simulink model "MagneticBasket_Simscape_Optimizer"  (R2023b)
settings: Solver=VariableStepAuto  StartTime=0.0  StopTime=SimParams.SimulationTime  MaxStep=1e-3
values from neighbouring files (symbols this model uses):
  m = obj.Br *obj.volume / obj.mu    [External_Magnet2.m]
  W = 1.5e-3    (= 0.0015)    [Sim_Open.m]
  x = x + link_length * sin(current_angle)    [Robot_Kinematics.m]    (also in Run_SimOpt.m = [Input.DipoleMoment_Angle{Input.Index} Input.DipoleMoment_Ma; magnetic_robot_simulation_old.m = x + dx; optimize_magnetic_robot.m = x + dx; optimize_magnetic_robot_second.m = x + dx)
undefined symbols (not defined in the file or in its folder): Fixed, magnet_HomePosition, SimParams, X, Y, Z
libraries: sm_lib x87, nesl_utility x48, vrlib x32, matrix_library x16
(part 3 of 3)

== system MagneticBasket_Simscape_Optimizer/Subsystem1/Magnetic Torque//Force Generator6 ==
  Calculate Magnetic Force/Torque : Subsystem
  Display{,1..4} (5 alike) : Display
  External Force and Torque : sm_lib/Forces and Torques/External Force and Torque  ForceResolutionFrame=AttachedFrame  EnableForceX=off  EnableForceY=off  EnableForceZ=off  EnableForce=on  TorqueResolutionFrame=AttachedFrame  EnableTorqueX=off  EnableTorqueY=off  EnableTorqueZ=off  EnableTorque=on
  Gain1 : Gain  Gain=SimParams.force_onoff
  Gain2 : Gain  Gain=SimParams.torque_onoff
  Indexing Needed : Gain  Gain=x(13)
  Indexing Needed2 : sm_lib/Frames and Transforms/Rigid Transform  TranslationMethod=None  TranslationStandardOffset=0  TranslationStandardOffsetUnits=m  TranslationStandardAxis=+Z  TranslationCartesianOffset=[0 0 0]  TranslationCartesianOffsetUnits=m  TranslationROffset=0  TranslationROffsetUnits=m  TranslationZOffset=0  TranslationZOffsetUnits=m  TranslationThetaOffset=0  TranslationThetaOffsetUnits=deg  RotationMethod=StandardAxis  RotationAngleUnits=deg  RotationStandardAxis=-Y  RotationAngle=x(6)*180/pi-90  RotationArbitraryAxis=[0 0 1]  FollAlignAxisA=+X  BaseAlignAxisA=+Y  FollAlignAxisB=+Y  BaseAlignAxisB=+Z  RotationSequenceAxes=FollowerAxes  RotationSequence=YXZ  RotationSequenceAngles=[-90 -90 0]  RotationSequenceAnglesUnits=deg  RotationMatrix=[1 0 0; 0 1 0; 0 0 1]  Quaternion=[1 0 0 0]
  Indexing Needed3 : sm_lib/Body Elements/Cylindrical Solid  GraphicAmbientColor=[0.15 0.15 0.15 1.0]  BasedOnType=Density  CenterOfMass=[0 0 0]  CenterOfMassUnits=m  GraphicDiffuseColor=[1 0 0]  CylinderLength=1e4*SimParams.arrow_scale*x(13)  CylinderLengthUnits=mm  CylinderRadius=SimParams.arrow_scale*0.05  CylinderRadiusUnits=mm  Density=0  DensityUnits=kg/m^3  DoExposeReferenceFrame=off  GraphicEmissiveColor=[0.0 0.0 0.0 1.0]  ExportEntireGeometry=off  SerializedFrames=<Frames><Frame><Id>Frame1</Id><Value><Name>F1</Name><Origin><Source>GeometricFeature</Source><FeatureName>top surface</FeatureName></Origin><PrimaryAxis><DefinedDirection>+Z</DefinedDirection><Source>ReferenceFrame</Source><SourceDirection>+Z</SourceDirection><FeatureName></FeatureName></PrimaryAxis><SecondaryAxis><DefinedDirection>+X</DefinedDirection><Source>ReferenceFrame</Source><SourceDirection>+X</SourceDirection><FeatureName></FeatureName></SecondaryAxis></Value></Frame><Frame><Id>Frame2</Id><Value><Name>F2</Name><Origin><Source>GeometricFeature</Source><FeatureName>bottom surface</FeatureName></Origin><PrimaryAxis><DefinedDirection>+Z</DefinedDirection><Source>ReferenceFrame</Source><SourceDirection>+Z</SourceDirection><FeatureName></FeatureName></PrimaryAxis><SecondaryAxis><DefinedDirection>+X</DefinedDirection><Source>ReferenceFrame</Source><SourceDirection>+X</SourceDirection><FeatureName></FeatureName></SecondaryAxis></Value></Frame></Frames>  MarkerShape=Sphere  MarkerSize=10  GraphicType=FromGeometry  InertiaType=CalculateFromGeometry  Mass=1  MassUnits=kg  MomentsOfInertia=[1 1 1]  MomentsOfInertiaUnits=kg*m^2  GraphicOpacity=SimParams.arrow_Opacity  ProductsOfInertia=[0 0 0]  ProductsOfInertiaUnits=kg*m^2  GraphicShininess=75  GraphicSpecularColor=[0.5 0.5 0.5 1.0]  GraphicVisPropType=SimpleVisualProperties
  Magnet DipoleMoment : Constant  Value=[Fixed.MagnetDirection 0]*Fixed.MagnetMagnitude
  MatrixMultiply : Product  Multiplication=Matrix(*)
  Normalize Vector : vrlib/Utilities/Normalize Vector  maxzero=0
  PS-Simulink Converter1 : nesl_utility/PS-Simulink Converter  PhysicalDomain=network_engine_domain  SubClassName=ps_output  LeftPortType=input  RightPortType=output  PseudoPeriodic=off  Frequencies=[]  VectorFormat=inherit  Unit=inherit  AffineConversion=off
  PS-Simulink Converter2 : nesl_utility/PS-Simulink Converter  PhysicalDomain=network_engine_domain  SubClassName=ps_output  LeftPortType=input  RightPortType=output  PseudoPeriodic=off  Frequencies=[]  VectorFormat=inherit  Unit=inherit  AffineConversion=off
  PS-Simulink Converter3 : nesl_utility/PS-Simulink Converter  PhysicalDomain=network_engine_domain  SubClassName=ps_output  LeftPortType=input  RightPortType=output  PseudoPeriodic=off  Frequencies=[]  VectorFormat=inherit  Unit=inherit  AffineConversion=off
  Revolved Solid : sm_lib/Body Elements/Revolved Solid  GraphicAmbientColor=[0.15 0.15 0.15 1.0]  BasedOnType=Density  CenterOfMass=[0 0 0]  CenterOfMassUnits=m  GraphicDiffuseColor=[1.0 0.0 0]  ExportConvexHullGeometry=off  Density=0  DensityUnits=kg/m^3  DoExposeReferenceFrame=on  GraphicEmissiveColor=[0.0 0.0 0.0 1.0]  ExportEntireGeometry=off  SerializedFrames=<Frames/>  MarkerShape=Sphere  MarkerSize=10  GraphicType=FromGeometry  InertiaType=CalculateFromGeometry  Mass=1  MassUnits=kg  MomentsOfInertia=[1 1 1]  MomentsOfInertiaUnits=kg*m^2  GraphicOpacity=SimParams.arrow_Opacity  ProductsOfInertia=[0 0 0]  ProductsOfInertiaUnits=kg*m^2  RevolutionCrossSection=[0 100; 0 0; 50 0]*SimParams.arrow_scale * 0.0025  RevolutionCrossSectionUnits=mm  RevolutionAngle=180  RevolutionAngleUnits=deg  RevolutionExtent=Full  GraphicShininess=75  GraphicSpecularColor=[0.5 0.5 0.5 1.0]  GraphicVisPropType=SimpleVisualProperties
  Simulink-PS Converter : nesl_utility/Simulink-PS Converter  PhysicalDomain=network_engine_domain  SubClassName=ps_input  LeftPortType=input  RightPortType=output  PseudoPeriodic=off  Frequencies=[]  NoiseDistribution=none  NoiseParameters=[]  Unit=1  AffineConversion=off  FilteringAndDerivatives=provide  SimscapeFilterOrder=1  InputFilterTimeConstant=0.001  UdotUserProvided=0
  Simulink-PS Converter1 : nesl_utility/Simulink-PS Converter  PhysicalDomain=network_engine_domain  SubClassName=ps_input  LeftPortType=input  RightPortType=output  PseudoPeriodic=off  Frequencies=[]  NoiseDistribution=none  NoiseParameters=[]  Unit=1  AffineConversion=off  FilteringAndDerivatives=provide  SimscapeFilterOrder=1  InputFilterTimeConstant=0.001  UdotUserProvided=0
  Submatrix1 : matrix_library/Submatrix  RowSpan=Range of rows  RowStartMode=First  RowStartIndex=1  RowEndMode=Last  RowEndIndex=1  ColSpan=One column  ColStartMode=Last  ColStartIndex=1  ColEndMode=Last  ColEndIndex=1
  Transform Sensor : sm_lib/Frames and Transforms/Transform Sensor  MeasurementFrame=World  RotationSequence=XYX  SenseAngle=off  SenseAxis=off  SenseQ=off  SenseR=off  SenseRotationSequence=off  SenseOmegaX=off  SenseOmegaY=off  SenseOmegaZ=off  SenseOmega=off  SenseQDot=off  SenseRDot=off  SenseRotationSequenceDot=off  SenseAlphaX=off  SenseAlphaY=off  SenseAlphaZ=off  SenseAlpha=off  SenseQDDot=off  SenseRDDot=off  SenseX=off  SenseY=off  SenseZ=off  SenseXYZ=on  SenseRad=off  SenseAzim=off  SenseDist=off  SenseInc=off  SenseXDot=off  SenseYDot=off  SenseZDot=off  SenseXYZDot=off  SenseRadDot=off  SenseAzimDot=off  SenseDistDot=off  SenseIncDot=off  SenseXDDot=off  SenseYDDot=off  SenseZDDot=off  SenseXYZDDot=off  SenseRadDDot=off  SenseAzimDDot=off  SenseDistDDot=off  SenseIncDDot=off
  Transform Sensor1 : sm_lib/Frames and Transforms/Transform Sensor  MeasurementFrame=Base  RotationSequence=XYX  SenseAngle=off  SenseAxis=off  SenseQ=off  SenseR=on  SenseRotationSequence=off  SenseOmegaX=off  SenseOmegaY=off  SenseOmegaZ=off  SenseOmega=off  SenseQDot=off  SenseRDot=off  SenseRotationSequenceDot=off  SenseAlphaX=off  SenseAlphaY=off  SenseAlphaZ=off  SenseAlpha=off  SenseQDDot=off  SenseRDDot=off  SenseX=off  SenseY=off  SenseZ=off  SenseXYZ=off  SenseRad=off  SenseAzim=off  SenseDist=off  SenseInc=off  SenseXDot=off  SenseYDot=off  SenseZDot=off  SenseXYZDot=off  SenseRadDot=off  SenseAzimDot=off  SenseDistDot=off  SenseIncDot=off  SenseXDDot=off  SenseYDDot=off  SenseZDDot=off  SenseXYZDDot=off  SenseRadDDot=off  SenseAzimDDot=off  SenseDistDDot=off  SenseIncDDot=off
  Transform Sensor2 : sm_lib/Frames and Transforms/Transform Sensor  MeasurementFrame=Base  RotationSequence=XYX  SenseAngle=off  SenseAxis=off  SenseQ=off  SenseR=on  SenseRotationSequence=off  SenseOmegaX=off  SenseOmegaY=off  SenseOmegaZ=off  SenseOmega=off  SenseQDot=off  SenseRDot=off  SenseRotationSequenceDot=off  SenseAlphaX=off  SenseAlphaY=off  SenseAlphaZ=off  SenseAlpha=off  SenseQDDot=off  SenseRDDot=off  SenseX=off  SenseY=off  SenseZ=off  SenseXYZ=off  SenseRad=off  SenseAzim=off  SenseDist=off  SenseInc=off  SenseXDot=off  SenseYDot=off  SenseZDot=off  SenseXYZDot=off  SenseRadDot=off  SenseAzimDot=off  SenseDistDot=off  SenseIncDot=off  SenseXDDot=off  SenseYDDot=off  SenseZDDot=off  SenseXYZDDot=off  SenseRadDDot=off  SenseAzimDDot=off  SenseDistDDot=off  SenseIncDDot=off
  Transpose : Math  Operator=transpose
  Magnet Frame : PMIOPort  Side=Left
  Plate Frame : PMIOPort  Port=2  Side=Right
  World Frame : PMIOPort  Port=3  Side=Left
  wires:
  Normalize Vector/1 -> Display2/1
  Gain1/1 -> Display4/1, Simulink-PS Converter/1
  Gain2/1 -> Display3/1, Simulink-PS Converter1/1
  PS-Simulink Converter2/1 -> Submatrix1/1
  Submatrix1/1 -> Indexing Needed/1
  PS-Simulink Converter1/1 -> Calculate Magnetic Force/Torque/2(r), Display1/1
  Magnet DipoleMoment/1 -> Calculate Magnetic Force/Torque/1(m1)  "world에서 본 뱡향"
  Indexing Needed/1 -> Display/1, Normalize Vector/1, Calculate Magnetic Force/Torque/3(m2)  "world에서 본 뱡향"
  Calculate Magnetic Force/Torque/1(Force) -> Gain1/1
  Calculate Magnetic Force/Torque/2(Torque) -> MatrixMultiply/2
  PS-Simulink Converter3/1 -> Transpose/1
  MatrixMultiply/1 -> Gain2/1
  Transpose/1 -> MatrixMultiply/1
  connections:
  Transform Sensor/LConn1 -- Magnet Frame/RConn1
  Indexing Needed2/RConn1 -- Indexing Needed3/RConn1 -- Transform Sensor1/RConn1 -- Transform Sensor/RConn1
  PS-Simulink Converter1/LConn1 -- Transform Sensor/RConn2
  Indexing Needed3/LConn1 -- Revolved Solid/RConn1
  Plate Frame/RConn1 -- Indexing Needed2/LConn1 -- External Force and Torque/RConn1 -- Transform Sensor2/RConn1
  External Force and Torque/LConn1 -- Simulink-PS Converter/RConn1
  Simulink-PS Converter1/RConn1 -- External Force and Torque/LConn2
  Transform Sensor1/LConn1 -- World Frame/RConn1 -- Transform Sensor2/LConn1
  PS-Simulink Converter2/LConn1 -- Transform Sensor1/RConn2
  PS-Simulink Converter3/LConn1 -- Transform Sensor2/RConn2

== system MagneticBasket_Simscape_Optimizer/Subsystem1/Magnetic Torque//Force Generator7 ==
  Calculate Magnetic Force/Torque : Subsystem
  Display{,1..4} (5 alike) : Display
  External Force and Torque : sm_lib/Forces and Torques/External Force and Torque  ForceResolutionFrame=AttachedFrame  EnableForceX=off  EnableForceY=off  EnableForceZ=off  EnableForce=on  TorqueResolutionFrame=AttachedFrame  EnableTorqueX=off  EnableTorqueY=off  EnableTorqueZ=off  EnableTorque=on
  Gain1 : Gain  Gain=SimParams.force_onoff
  Gain2 : Gain  Gain=SimParams.torque_onoff
  Indexing Needed : Gain  Gain=x(14)
  Indexing Needed2 : sm_lib/Frames and Transforms/Rigid Transform  TranslationMethod=None  TranslationStandardOffset=0  TranslationStandardOffsetUnits=m  TranslationStandardAxis=+Z  TranslationCartesianOffset=[0 0 0]  TranslationCartesianOffsetUnits=m  TranslationROffset=0  TranslationROffsetUnits=m  TranslationZOffset=0  TranslationZOffsetUnits=m  TranslationThetaOffset=0  TranslationThetaOffsetUnits=deg  RotationMethod=StandardAxis  RotationAngleUnits=deg  RotationStandardAxis=-Y  RotationAngle=x(7)*180/pi-90  RotationArbitraryAxis=[0 0 1]  FollAlignAxisA=+X  BaseAlignAxisA=+Y  FollAlignAxisB=+Y  BaseAlignAxisB=+Z  RotationSequenceAxes=FollowerAxes  RotationSequence=YXZ  RotationSequenceAngles=[-90 -90 0]  RotationSequenceAnglesUnits=deg  RotationMatrix=[1 0 0; 0 1 0; 0 0 1]  Quaternion=[1 0 0 0]
  Indexing Needed3 : sm_lib/Body Elements/Cylindrical Solid  GraphicAmbientColor=[0.15 0.15 0.15 1.0]  BasedOnType=Density  CenterOfMass=[0 0 0]  CenterOfMassUnits=m  GraphicDiffuseColor=[1 0 0]  CylinderLength=1e4*SimParams.arrow_scale*x(14)  CylinderLengthUnits=mm  CylinderRadius=SimParams.arrow_scale*0.05  CylinderRadiusUnits=mm  Density=0  DensityUnits=kg/m^3  DoExposeReferenceFrame=off  GraphicEmissiveColor=[0.0 0.0 0.0 1.0]  ExportEntireGeometry=off  SerializedFrames=<Frames><Frame><Id>Frame1</Id><Value><Name>F1</Name><Origin><Source>GeometricFeature</Source><FeatureName>top surface</FeatureName></Origin><PrimaryAxis><DefinedDirection>+Z</DefinedDirection><Source>ReferenceFrame</Source><SourceDirection>+Z</SourceDirection><FeatureName></FeatureName></PrimaryAxis><SecondaryAxis><DefinedDirection>+X</DefinedDirection><Source>ReferenceFrame</Source><SourceDirection>+X</SourceDirection><FeatureName></FeatureName></SecondaryAxis></Value></Frame><Frame><Id>Frame2</Id><Value><Name>F2</Name><Origin><Source>GeometricFeature</Source><FeatureName>bottom surface</FeatureName></Origin><PrimaryAxis><DefinedDirection>+Z</DefinedDirection><Source>ReferenceFrame</Source><SourceDirection>+Z</SourceDirection><FeatureName></FeatureName></PrimaryAxis><SecondaryAxis><DefinedDirection>+X</DefinedDirection><Source>ReferenceFrame</Source><SourceDirection>+X</SourceDirection><FeatureName></FeatureName></SecondaryAxis></Value></Frame></Frames>  MarkerShape=Sphere  MarkerSize=10  GraphicType=FromGeometry  InertiaType=CalculateFromGeometry  Mass=1  MassUnits=kg  MomentsOfInertia=[1 1 1]  MomentsOfInertiaUnits=kg*m^2  GraphicOpacity=SimParams.arrow_Opacity  ProductsOfInertia=[0 0 0]  ProductsOfInertiaUnits=kg*m^2  GraphicShininess=75  GraphicSpecularColor=[0.5 0.5 0.5 1.0]  GraphicVisPropType=SimpleVisualProperties
  Magnet DipoleMoment : Constant  Value=[Fixed.MagnetDirection 0]*Fixed.MagnetMagnitude
  MatrixMultiply : Product  Multiplication=Matrix(*)
  Normalize Vector : vrlib/Utilities/Normalize Vector  maxzero=0
  PS-Simulink Converter1 : nesl_utility/PS-Simulink Converter  PhysicalDomain=network_engine_domain  SubClassName=ps_output  LeftPortType=input  RightPortType=output  PseudoPeriodic=off  Frequencies=[]  VectorFormat=inherit  Unit=inherit  AffineConversion=off
  PS-Simulink Converter2 : nesl_utility/PS-Simulink Converter  PhysicalDomain=network_engine_domain  SubClassName=ps_output  LeftPortType=input  RightPortType=output  PseudoPeriodic=off  Frequencies=[]  VectorFormat=inherit  Unit=inherit  AffineConversion=off
  PS-Simulink Converter3 : nesl_utility/PS-Simulink Converter  PhysicalDomain=network_engine_domain  SubClassName=ps_output  LeftPortType=input  RightPortType=output  PseudoPeriodic=off  Frequencies=[]  VectorFormat=inherit  Unit=inherit  AffineConversion=off
  Revolved Solid : sm_lib/Body Elements/Revolved Solid  GraphicAmbientColor=[0.15 0.15 0.15 1.0]  BasedOnType=Density  CenterOfMass=[0 0 0]  CenterOfMassUnits=m  GraphicDiffuseColor=[1.0 0.0 0]  ExportConvexHullGeometry=off  Density=0  DensityUnits=kg/m^3  DoExposeReferenceFrame=on  GraphicEmissiveColor=[0.0 0.0 0.0 1.0]  ExportEntireGeometry=off  SerializedFrames=<Frames/>  MarkerShape=Sphere  MarkerSize=10  GraphicType=FromGeometry  InertiaType=CalculateFromGeometry  Mass=1  MassUnits=kg  MomentsOfInertia=[1 1 1]  MomentsOfInertiaUnits=kg*m^2  GraphicOpacity=SimParams.arrow_Opacity  ProductsOfInertia=[0 0 0]  ProductsOfInertiaUnits=kg*m^2  RevolutionCrossSection=[0 100; 0 0; 50 0]*SimParams.arrow_scale * 0.0025  RevolutionCrossSectionUnits=mm  RevolutionAngle=180  RevolutionAngleUnits=deg  RevolutionExtent=Full  GraphicShininess=75  GraphicSpecularColor=[0.5 0.5 0.5 1.0]  GraphicVisPropType=SimpleVisualProperties
  Simulink-PS Converter : nesl_utility/Simulink-PS Converter  PhysicalDomain=network_engine_domain  SubClassName=ps_input  LeftPortType=input  RightPortType=output  PseudoPeriodic=off  Frequencies=[]  NoiseDistribution=none  NoiseParameters=[]  Unit=1  AffineConversion=off  FilteringAndDerivatives=provide  SimscapeFilterOrder=1  InputFilterTimeConstant=0.001  UdotUserProvided=0
  Simulink-PS Converter1 : nesl_utility/Simulink-PS Converter  PhysicalDomain=network_engine_domain  SubClassName=ps_input  LeftPortType=input  RightPortType=output  PseudoPeriodic=off  Frequencies=[]  NoiseDistribution=none  NoiseParameters=[]  Unit=1  AffineConversion=off  FilteringAndDerivatives=provide  SimscapeFilterOrder=1  InputFilterTimeConstant=0.001  UdotUserProvided=0
  Submatrix1 : matrix_library/Submatrix  RowSpan=Range of rows  RowStartMode=First  RowStartIndex=1  RowEndMode=Last  RowEndIndex=1  ColSpan=One column  ColStartMode=Last  ColStartIndex=1  ColEndMode=Last  ColEndIndex=1
  Transform Sensor : sm_lib/Frames and Transforms/Transform Sensor  MeasurementFrame=World  RotationSequence=XYX  SenseAngle=off  SenseAxis=off  SenseQ=off  SenseR=off  SenseRotationSequence=off  SenseOmegaX=off  SenseOmegaY=off  SenseOmegaZ=off  SenseOmega=off  SenseQDot=off  SenseRDot=off  SenseRotationSequenceDot=off  SenseAlphaX=off  SenseAlphaY=off  SenseAlphaZ=off  SenseAlpha=off  SenseQDDot=off  SenseRDDot=off  SenseX=off  SenseY=off  SenseZ=off  SenseXYZ=on  SenseRad=off  SenseAzim=off  SenseDist=off  SenseInc=off  SenseXDot=off  SenseYDot=off  SenseZDot=off  SenseXYZDot=off  SenseRadDot=off  SenseAzimDot=off  SenseDistDot=off  SenseIncDot=off  SenseXDDot=off  SenseYDDot=off  SenseZDDot=off  SenseXYZDDot=off  SenseRadDDot=off  SenseAzimDDot=off  SenseDistDDot=off  SenseIncDDot=off
  Transform Sensor1 : sm_lib/Frames and Transforms/Transform Sensor  MeasurementFrame=Base  RotationSequence=XYX  SenseAngle=off  SenseAxis=off  SenseQ=off  SenseR=on  SenseRotationSequence=off  SenseOmegaX=off  SenseOmegaY=off  SenseOmegaZ=off  SenseOmega=off  SenseQDot=off  SenseRDot=off  SenseRotationSequenceDot=off  SenseAlphaX=off  SenseAlphaY=off  SenseAlphaZ=off  SenseAlpha=off  SenseQDDot=off  SenseRDDot=off  SenseX=off  SenseY=off  SenseZ=off  SenseXYZ=off  SenseRad=off  SenseAzim=off  SenseDist=off  SenseInc=off  SenseXDot=off  SenseYDot=off  SenseZDot=off  SenseXYZDot=off  SenseRadDot=off  SenseAzimDot=off  SenseDistDot=off  SenseIncDot=off  SenseXDDot=off  SenseYDDot=off  SenseZDDot=off  SenseXYZDDot=off  SenseRadDDot=off  SenseAzimDDot=off  SenseDistDDot=off  SenseIncDDot=off
  Transform Sensor2 : sm_lib/Frames and Transforms/Transform Sensor  MeasurementFrame=Base  RotationSequence=XYX  SenseAngle=off  SenseAxis=off  SenseQ=off  SenseR=on  SenseRotationSequence=off  SenseOmegaX=off  SenseOmegaY=off  SenseOmegaZ=off  SenseOmega=off  SenseQDot=off  SenseRDot=off  SenseRotationSequenceDot=off  SenseAlphaX=off  SenseAlphaY=off  SenseAlphaZ=off  SenseAlpha=off  SenseQDDot=off  SenseRDDot=off  SenseX=off  SenseY=off  SenseZ=off  SenseXYZ=off  SenseRad=off  SenseAzim=off  SenseDist=off  SenseInc=off  SenseXDot=off  SenseYDot=off  SenseZDot=off  SenseXYZDot=off  SenseRadDot=off  SenseAzimDot=off  SenseDistDot=off  SenseIncDot=off  SenseXDDot=off  SenseYDDot=off  SenseZDDot=off  SenseXYZDDot=off  SenseRadDDot=off  SenseAzimDDot=off  SenseDistDDot=off  SenseIncDDot=off
  Transpose : Math  Operator=transpose
  Magnet Frame : PMIOPort  Side=Left
  Plate Frame : PMIOPort  Port=2  Side=Right
  World Frame : PMIOPort  Port=3  Side=Left
  wires:
  Transpose/1 -> MatrixMultiply/1
  MatrixMultiply/1 -> Gain2/1
  PS-Simulink Converter3/1 -> Transpose/1
  Calculate Magnetic Force/Torque/2(Torque) -> MatrixMultiply/2
  Calculate Magnetic Force/Torque/1(Force) -> Display4/1, Gain1/1
  Indexing Needed/1 -> Calculate Magnetic Force/Torque/3(m2), Normalize Vector/1, Display/1  "world에서 본 뱡향"
  Magnet DipoleMoment/1 -> Calculate Magnetic Force/Torque/1(m1)  "world에서 본 뱡향"
  PS-Simulink Converter1/1 -> Display1/1, Calculate Magnetic Force/Torque/2(r)
  Submatrix1/1 -> Indexing Needed/1
  PS-Simulink Converter2/1 -> Submatrix1/1
  Gain2/1 -> Simulink-PS Converter1/1, Display3/1
  Gain1/1 -> Simulink-PS Converter/1
  Normalize Vector/1 -> Display2/1
  connections:
  PS-Simulink Converter3/LConn1 -- Transform Sensor2/RConn2
  PS-Simulink Converter2/LConn1 -- Transform Sensor1/RConn2
  Transform Sensor2/LConn1 -- World Frame/RConn1 -- Transform Sensor1/LConn1
  Simulink-PS Converter1/RConn1 -- External Force and Torque/LConn2
  External Force and Torque/LConn1 -- Simulink-PS Converter/RConn1
  Transform Sensor2/RConn1 -- External Force and Torque/RConn1 -- Indexing Needed2/LConn1 -- Plate Frame/RConn1
  Indexing Needed3/LConn1 -- Revolved Solid/RConn1
  PS-Simulink Converter1/LConn1 -- Transform Sensor/RConn2
  Transform Sensor/RConn1 -- Transform Sensor1/RConn1 -- Indexing Needed3/RConn1 -- Indexing Needed2/RConn1
  Transform Sensor/LConn1 -- Magnet Frame/RConn1

== system MagneticBasket_Simscape_Optimizer/Magnetic Torque//Force Generator StartPlane/Calculate Magnetic Force//Torque/Magnetic Force ==
  r : Inport
  m1 : Inport  Port=2
  m2 : Inport  Port=3
  Add : Sum  Inputs=+++
  Add2 : Sum  Inputs=+-
  Constant : Constant  Value=-4
  Display : Display
  Dot Product{1..5} (5 alike) : DotProduct  OutDataTypeStr=Inherit: Inherit via internal rule
  Gain : Gain  Gain=5
  Gain3 : Gain  Gain=3*Fixed.myu/(4*pi)
  Normalize Vector : vrlib/Utilities/Normalize Vector  maxzero=0
  Power : Math  Operator=pow
  Product{,1,4,6} (4 alike) : Product
  Sqrt : Sqrt
  Force : Outport
  wires:
  Sqrt/1 -> Power/1
  Product/1 -> Display/1, Add/3
  Add2/1 -> Product/2
  Add/1 -> Product4/2
  Product6/1 -> Add/1
  Product1/1 -> Add/2
  Gain/1 -> Add2/2  "5 * dot(m1,r_hat) * dot(m2,r_hat)"
  Dot Product5/1 -> Gain/1
  Dot Product3/1 -> Add2/1  "dot(m1,m2)"
  Dot Product2/1 -> Dot Product5/2, Product1/1  "dot(m2,r_hat)"
  Dot Product4/1 -> Dot Product5/1, Product6/1  "dot(m1,r_hat)"
  m2/1 -> Product6/2, Dot Product2/2, Dot Product3/2  "m2"
  m1/1 -> Dot Product4/2, Product1/2, Dot Product3/1  "m1"
  Normalize Vector/1 -> Dot Product4/1, Dot Product2/1, Product/1  "r_hat"
  r/1 -> Dot Product1/1, Dot Product1/2, Normalize Vector/1
  Product4/1 -> Force/1
  Gain3/1 -> Product4/1  "3*myu_0/(4*pi*r^4)"
  Power/1 -> Gain3/1
  Constant/1 -> Power/2
  Dot Product1/1 -> Sqrt/1

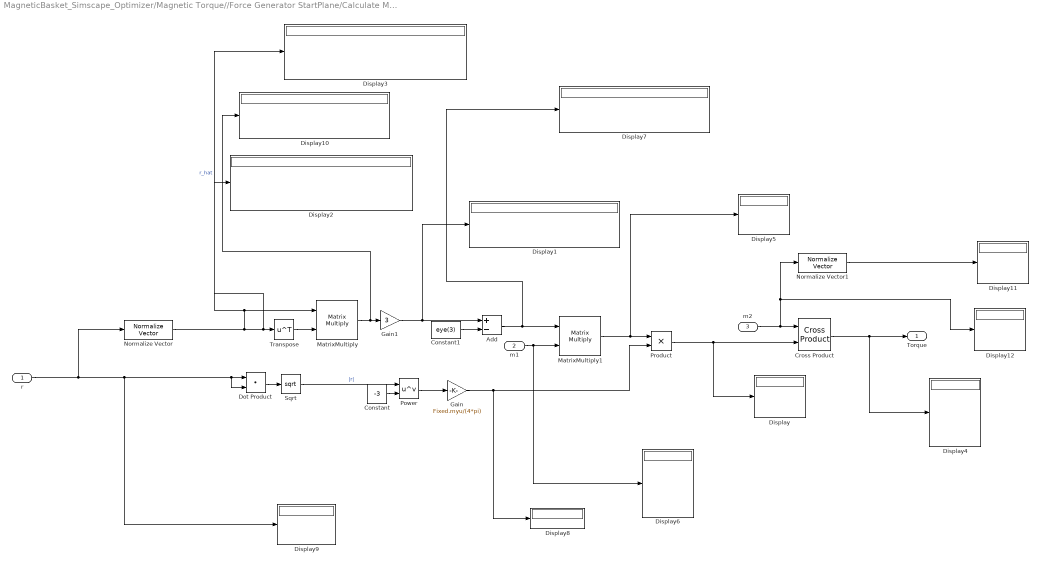
== system MagneticBasket_Simscape_Optimizer/Magnetic Torque//Force Generator StartPlane/Calculate Magnetic Force//Torque/Magnetic Torque ==
  r : Inport
  m1 : Inport  Port=2
  m2 : Inport  Port=3
  Add : Sum  Inputs=+-
  Constant : Constant  Value=-3
  Constant1 : Constant  Value=eye(3)
  Cross Product : matrix_library/Cross Product
  Display{,1..12} (13 alike) : Display
  Dot Product : DotProduct  OutDataTypeStr=Inherit: Inherit via internal rule
  Gain : Gain  Gain=Fixed.myu/(4*pi)
  Gain1 : Gain  Gain=3
  MatrixMultiply : Product  Multiplication=Matrix(*)
  MatrixMultiply1 : Product  Multiplication=Matrix(*)
  Normalize Vector : vrlib/Utilities/Normalize Vector  maxzero=0
  Normalize Vector1 : vrlib/Utilities/Normalize Vector  maxzero=0
  Power : Math  Operator=pow
  Product : Product
  Sqrt : Sqrt
  Transpose : Math  Operator=transpose
  Torque : Outport
  wires:
  Normalize Vector1/1 -> Display11/1
  Sqrt/1 -> Power/1  "|r|"
  Gain1/1 -> Display1/1, Add/1
  Product/1 -> Cross Product/2, Display/1
  MatrixMultiply1/1 -> Product/1, Display5/1
  Gain/1 -> Product/2, Display8/1
  m1/1 -> MatrixMultiply1/2, Display6/1
  Add/1 -> MatrixMultiply1/1, Display7/1
  Constant1/1 -> Add/2
  MatrixMultiply/1 -> Gain1/1, Display10/1
  Transpose/1 -> MatrixMultiply/2
  Normalize Vector/1 -> Display2/1, MatrixMultiply/1, Transpose/1, Display3/1  "r_hat"
  Power/1 -> Gain/1
  Constant/1 -> Power/2
  Dot Product/1 -> Sqrt/1
  r/1 -> Normalize Vector/1, Dot Product/1, Dot Product/2, Display9/1
  m2/1 -> Cross Product/1, Normalize Vector1/1, Display12/1
  Cross Product/1 -> Torque/1, Display4/1

== system MagneticBasket_Simscape_Optimizer/Subsystem1/Magnetic Torque//Force Generator1/Calculate Magnetic Force//Torque ==
  m1 : Inport
  r : Inport  Port=2
  m2 : Inport  Port=3
  Magnetic Force : Subsystem
  Magnetic Torque : Subsystem
  Force : Outport
  Torque : Outport  Port=2
  wires:
  Magnetic Force/1(Force) -> Force/1
  Magnetic Torque/1(Torque) -> Torque/1
  r/1 -> Magnetic Torque/1(r), Magnetic Force/1(r)
  m2/1 -> Magnetic Torque/3(m2), Magnetic Force/3(m2)
  m1/1 -> Magnetic Torque/2(m1), Magnetic Force/2(m1)

== system MagneticBasket_Simscape_Optimizer/Subsystem1/Magnetic Torque//Force Generator2/Calculate Magnetic Force//Torque ==
  m1 : Inport
  r : Inport  Port=2
  m2 : Inport  Port=3
  Magnetic Force : Subsystem
  Magnetic Torque : Subsystem
  Force : Outport
  Torque : Outport  Port=2
  wires:
  m1/1 -> Magnetic Force/2(m1), Magnetic Torque/2(m1)
  m2/1 -> Magnetic Force/3(m2), Magnetic Torque/3(m2)
  r/1 -> Magnetic Force/1(r), Magnetic Torque/1(r)
  Magnetic Torque/1(Torque) -> Torque/1
  Magnetic Force/1(Force) -> Force/1

== system MagneticBasket_Simscape_Optimizer/Subsystem1/Magnetic Torque//Force Generator3/Calculate Magnetic Force//Torque ==
  m1 : Inport
  r : Inport  Port=2
  m2 : Inport  Port=3
  Magnetic Force : Subsystem
  Magnetic Torque : Subsystem
  Force : Outport
  Torque : Outport  Port=2
  wires:
  Magnetic Force/1(Force) -> Force/1
  Magnetic Torque/1(Torque) -> Torque/1
  r/1 -> Magnetic Torque/1(r), Magnetic Force/1(r)
  m2/1 -> Magnetic Torque/3(m2), Magnetic Force/3(m2)
  m1/1 -> Magnetic Torque/2(m1), Magnetic Force/2(m1)

== system MagneticBasket_Simscape_Optimizer/Subsystem1/Magnetic Torque//Force Generator4/Calculate Magnetic Force//Torque ==
  m1 : Inport
  r : Inport  Port=2
  m2 : Inport  Port=3
  Magnetic Force : Subsystem
  Magnetic Torque : Subsystem
  Force : Outport
  Torque : Outport  Port=2
  wires:
  m1/1 -> Magnetic Force/2(m1), Magnetic Torque/2(m1)
  m2/1 -> Magnetic Force/3(m2), Magnetic Torque/3(m2)
  r/1 -> Magnetic Force/1(r), Magnetic Torque/1(r)
  Magnetic Torque/1(Torque) -> Torque/1
  Magnetic Force/1(Force) -> Force/1

== system MagneticBasket_Simscape_Optimizer/Subsystem1/Magnetic Torque//Force Generator5/Calculate Magnetic Force//Torque ==
  m1 : Inport
  r : Inport  Port=2
  m2 : Inport  Port=3
  Magnetic Force : Subsystem
  Magnetic Torque : Subsystem
  Force : Outport
  Torque : Outport  Port=2
  wires:
  Magnetic Force/1(Force) -> Force/1
  Magnetic Torque/1(Torque) -> Torque/1
  r/1 -> Magnetic Torque/1(r), Magnetic Force/1(r)
  m2/1 -> Magnetic Torque/3(m2), Magnetic Force/3(m2)
  m1/1 -> Magnetic Torque/2(m1), Magnetic Force/2(m1)

== system MagneticBasket_Simscape_Optimizer/Subsystem1/Magnetic Torque//Force Generator6/Calculate Magnetic Force//Torque ==
  m1 : Inport
  r : Inport  Port=2
  m2 : Inport  Port=3
  Magnetic Force : Subsystem
  Magnetic Torque : Subsystem
  Force : Outport
  Torque : Outport  Port=2
  wires:
  m1/1 -> Magnetic Force/2(m1), Magnetic Torque/2(m1)
  m2/1 -> Magnetic Force/3(m2), Magnetic Torque/3(m2)
  r/1 -> Magnetic Force/1(r), Magnetic Torque/1(r)
  Magnetic Torque/1(Torque) -> Torque/1
  Magnetic Force/1(Force) -> Force/1

== system MagneticBasket_Simscape_Optimizer/Subsystem1/Magnetic Torque//Force Generator7/Calculate Magnetic Force//Torque ==
  m1 : Inport
  r : Inport  Port=2
  m2 : Inport  Port=3
  Magnetic Force : Subsystem
  Magnetic Torque : Subsystem
  Force : Outport
  Torque : Outport  Port=2
  wires:
  Magnetic Force/1(Force) -> Force/1
  Magnetic Torque/1(Torque) -> Torque/1
  r/1 -> Magnetic Torque/1(r), Magnetic Force/1(r)
  m2/1 -> Magnetic Torque/3(m2), Magnetic Force/3(m2)
  m1/1 -> Magnetic Torque/2(m1), Magnetic Force/2(m1)

== system MagneticBasket_Simscape_Optimizer/Subsystem1/Magnetic Torque//Force Generator1/Calculate Magnetic Force//Torque/Magnetic Force ==
  r : Inport
  m1 : Inport  Port=2
  m2 : Inport  Port=3
  Add : Sum  Inputs=+++
  Add2 : Sum  Inputs=+-
  Constant : Constant  Value=-4
  Display : Display
  Dot Product{1..5} (5 alike) : DotProduct  OutDataTypeStr=Inherit: Inherit via internal rule
  Gain : Gain  Gain=5
  Gain3 : Gain  Gain=3*Fixed.myu/(4*pi)
  Normalize Vector : vrlib/Utilities/Normalize Vector  maxzero=0
  Power : Math  Operator=pow
  Product{,1,4,6} (4 alike) : Product
  Sqrt : Sqrt
  Force : Outport
  wires:
  Sqrt/1 -> Power/1
  Product/1 -> Display/1, Add/3
  Add2/1 -> Product/2
  Add/1 -> Product4/2
  Product6/1 -> Add/1
  Product1/1 -> Add/2
  Gain/1 -> Add2/2  "5 * dot(m1,r_hat) * dot(m2,r_hat)"
  Dot Product5/1 -> Gain/1
  Dot Product3/1 -> Add2/1  "dot(m1,m2)"
  Dot Product2/1 -> Dot Product5/2, Product1/1  "dot(m2,r_hat)"
  Dot Product4/1 -> Dot Product5/1, Product6/1  "dot(m1,r_hat)"
  m2/1 -> Product6/2, Dot Product2/2, Dot Product3/2  "m2"
  m1/1 -> Dot Product4/2, Product1/2, Dot Product3/1  "m1"
  Normalize Vector/1 -> Dot Product4/1, Dot Product2/1, Product/1  "r_hat"
  r/1 -> Dot Product1/1, Dot Product1/2, Normalize Vector/1
  Product4/1 -> Force/1
  Gain3/1 -> Product4/1  "3*myu_0/(4*pi*r^4)"
  Power/1 -> Gain3/1
  Constant/1 -> Power/2
  Dot Product1/1 -> Sqrt/1

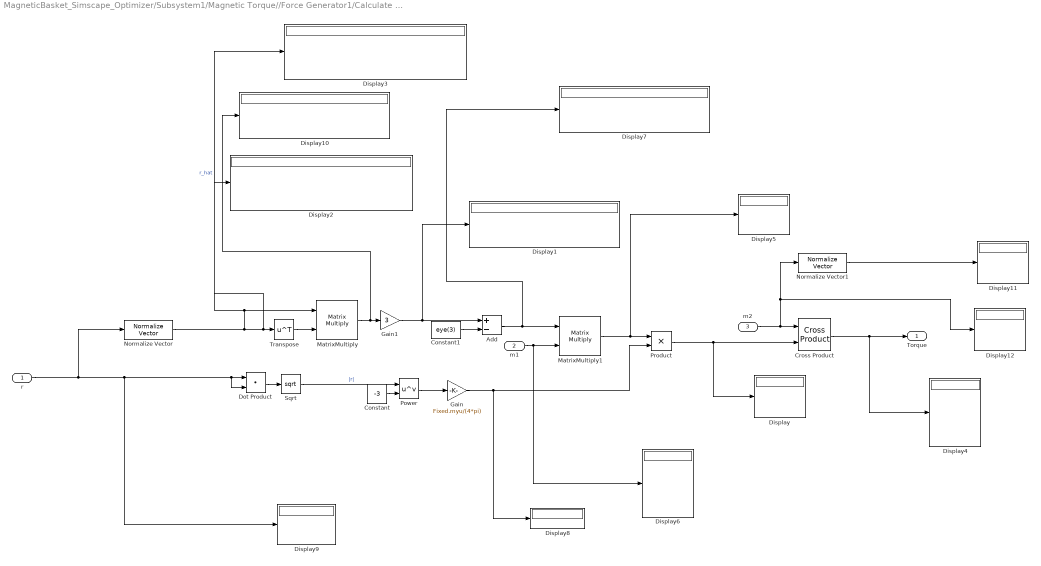
== system MagneticBasket_Simscape_Optimizer/Subsystem1/Magnetic Torque//Force Generator1/Calculate Magnetic Force//Torque/Magnetic Torque ==
  r : Inport
  m1 : Inport  Port=2
  m2 : Inport  Port=3
  Add : Sum  Inputs=+-
  Constant : Constant  Value=-3
  Constant1 : Constant  Value=eye(3)
  Cross Product : matrix_library/Cross Product
  Display{,1..12} (13 alike) : Display
  Dot Product : DotProduct  OutDataTypeStr=Inherit: Inherit via internal rule
  Gain : Gain  Gain=Fixed.myu/(4*pi)
  Gain1 : Gain  Gain=3
  MatrixMultiply : Product  Multiplication=Matrix(*)
  MatrixMultiply1 : Product  Multiplication=Matrix(*)
  Normalize Vector : vrlib/Utilities/Normalize Vector  maxzero=0
  Normalize Vector1 : vrlib/Utilities/Normalize Vector  maxzero=0
  Power : Math  Operator=pow
  Product : Product
  Sqrt : Sqrt
  Transpose : Math  Operator=transpose
  Torque : Outport
  wires:
  Normalize Vector1/1 -> Display11/1
  Sqrt/1 -> Power/1  "|r|"
  Gain1/1 -> Display1/1, Add/1
  Product/1 -> Cross Product/2, Display/1
  MatrixMultiply1/1 -> Product/1, Display5/1
  Gain/1 -> Product/2, Display8/1
  m1/1 -> MatrixMultiply1/2, Display6/1
  Add/1 -> MatrixMultiply1/1, Display7/1
  Constant1/1 -> Add/2
  MatrixMultiply/1 -> Gain1/1, Display10/1
  Transpose/1 -> MatrixMultiply/2
  Normalize Vector/1 -> Display2/1, MatrixMultiply/1, Transpose/1, Display3/1  "r_hat"
  Power/1 -> Gain/1
  Constant/1 -> Power/2
  Dot Product/1 -> Sqrt/1
  r/1 -> Normalize Vector/1, Dot Product/1, Dot Product/2, Display9/1
  m2/1 -> Cross Product/1, Normalize Vector1/1, Display12/1
  Cross Product/1 -> Torque/1, Display4/1

== system MagneticBasket_Simscape_Optimizer/Subsystem1/Magnetic Torque//Force Generator2/Calculate Magnetic Force//Torque/Magnetic Force ==
  r : Inport
  m1 : Inport  Port=2
  m2 : Inport  Port=3
  Add : Sum  Inputs=+++
  Add2 : Sum  Inputs=+-
  Constant : Constant  Value=-4
  Display : Display
  Dot Product{1..5} (5 alike) : DotProduct  OutDataTypeStr=Inherit: Inherit via internal rule
  Gain : Gain  Gain=5
  Gain3 : Gain  Gain=3*Fixed.myu/(4*pi)
  Normalize Vector : vrlib/Utilities/Normalize Vector  maxzero=0
  Power : Math  Operator=pow
  Product{,1,4,6} (4 alike) : Product
  Sqrt : Sqrt
  Force : Outport
  wires:
  Dot Product1/1 -> Sqrt/1
  Constant/1 -> Power/2
  Power/1 -> Gain3/1
  Gain3/1 -> Product4/1  "3*myu_0/(4*pi*r^4)"
  Product4/1 -> Force/1
  r/1 -> Normalize Vector/1, Dot Product1/2, Dot Product1/1
  Normalize Vector/1 -> Product/1, Dot Product2/1, Dot Product4/1  "r_hat"
  m1/1 -> Dot Product3/1, Product1/2, Dot Product4/2  "m1"
  m2/1 -> Dot Product3/2, Dot Product2/2, Product6/2  "m2"
  Dot Product4/1 -> Product6/1, Dot Product5/1  "dot(m1,r_hat)"
  Dot Product2/1 -> Product1/1, Dot Product5/2  "dot(m2,r_hat)"
  Dot Product3/1 -> Add2/1  "dot(m1,m2)"
  Dot Product5/1 -> Gain/1
  Gain/1 -> Add2/2  "5 * dot(m1,r_hat) * dot(m2,r_hat)"
  Product1/1 -> Add/2
  Product6/1 -> Add/1
  Add/1 -> Product4/2
  Add2/1 -> Product/2
  Product/1 -> Add/3, Display/1
  Sqrt/1 -> Power/1

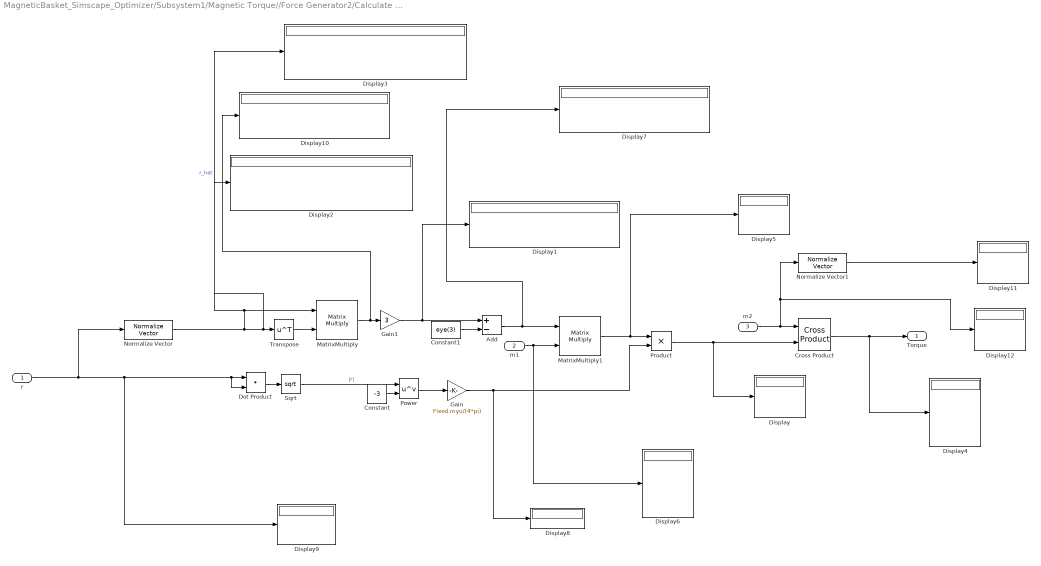
== system MagneticBasket_Simscape_Optimizer/Subsystem1/Magnetic Torque//Force Generator2/Calculate Magnetic Force//Torque/Magnetic Torque ==
  r : Inport
  m1 : Inport  Port=2
  m2 : Inport  Port=3
  Add : Sum  Inputs=+-
  Constant : Constant  Value=-3
  Constant1 : Constant  Value=eye(3)
  Cross Product : matrix_library/Cross Product
  Display{,1..12} (13 alike) : Display
  Dot Product : DotProduct  OutDataTypeStr=Inherit: Inherit via internal rule
  Gain : Gain  Gain=Fixed.myu/(4*pi)
  Gain1 : Gain  Gain=3
  MatrixMultiply : Product  Multiplication=Matrix(*)
  MatrixMultiply1 : Product  Multiplication=Matrix(*)
  Normalize Vector : vrlib/Utilities/Normalize Vector  maxzero=0
  Normalize Vector1 : vrlib/Utilities/Normalize Vector  maxzero=0
  Power : Math  Operator=pow
  Product : Product
  Sqrt : Sqrt
  Transpose : Math  Operator=transpose
  Torque : Outport
  wires:
  Cross Product/1 -> Display4/1, Torque/1
  m2/1 -> Display12/1, Normalize Vector1/1, Cross Product/1
  r/1 -> Display9/1, Dot Product/2, Dot Product/1, Normalize Vector/1
  Dot Product/1 -> Sqrt/1
  Constant/1 -> Power/2
  Power/1 -> Gain/1
  Normalize Vector/1 -> Display3/1, Transpose/1, MatrixMultiply/1, Display2/1  "r_hat"
  Transpose/1 -> MatrixMultiply/2
  MatrixMultiply/1 -> Display10/1, Gain1/1
  Constant1/1 -> Add/2
  Add/1 -> Display7/1, MatrixMultiply1/1
  m1/1 -> Display6/1, MatrixMultiply1/2
  Gain/1 -> Display8/1, Product/2
  MatrixMultiply1/1 -> Display5/1, Product/1
  Product/1 -> Display/1, Cross Product/2
  Gain1/1 -> Add/1, Display1/1
  Sqrt/1 -> Power/1  "|r|"
  Normalize Vector1/1 -> Display11/1

== system MagneticBasket_Simscape_Optimizer/Subsystem1/Magnetic Torque//Force Generator3/Calculate Magnetic Force//Torque/Magnetic Force ==
  r : Inport
  m1 : Inport  Port=2
  m2 : Inport  Port=3
  Add : Sum  Inputs=+++
  Add2 : Sum  Inputs=+-
  Constant : Constant  Value=-4
  Display : Display
  Dot Product{1..5} (5 alike) : DotProduct  OutDataTypeStr=Inherit: Inherit via internal rule
  Gain : Gain  Gain=5
  Gain3 : Gain  Gain=3*Fixed.myu/(4*pi)
  Normalize Vector : vrlib/Utilities/Normalize Vector  maxzero=0
  Power : Math  Operator=pow
  Product{,1,4,6} (4 alike) : Product
  Sqrt : Sqrt
  Force : Outport
  wires:
  Sqrt/1 -> Power/1
  Product/1 -> Display/1, Add/3
  Add2/1 -> Product/2
  Add/1 -> Product4/2
  Product6/1 -> Add/1
  Product1/1 -> Add/2
  Gain/1 -> Add2/2  "5 * dot(m1,r_hat) * dot(m2,r_hat)"
  Dot Product5/1 -> Gain/1
  Dot Product3/1 -> Add2/1  "dot(m1,m2)"
  Dot Product2/1 -> Dot Product5/2, Product1/1  "dot(m2,r_hat)"
  Dot Product4/1 -> Dot Product5/1, Product6/1  "dot(m1,r_hat)"
  m2/1 -> Product6/2, Dot Product2/2, Dot Product3/2  "m2"
  m1/1 -> Dot Product4/2, Product1/2, Dot Product3/1  "m1"
  Normalize Vector/1 -> Dot Product4/1, Dot Product2/1, Product/1  "r_hat"
  r/1 -> Dot Product1/1, Dot Product1/2, Normalize Vector/1
  Product4/1 -> Force/1
  Gain3/1 -> Product4/1  "3*myu_0/(4*pi*r^4)"
  Power/1 -> Gain3/1
  Constant/1 -> Power/2
  Dot Product1/1 -> Sqrt/1

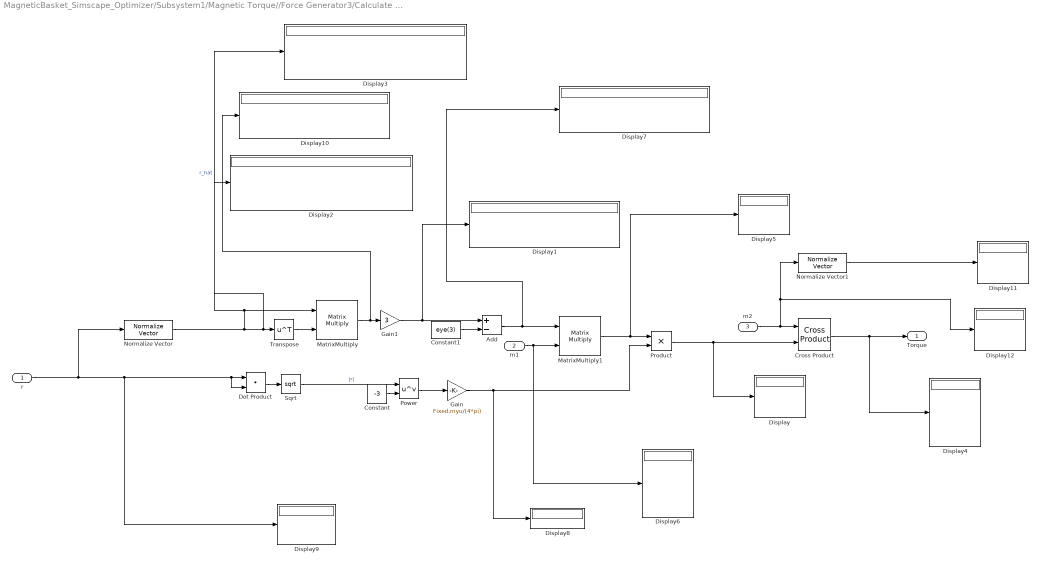
== system MagneticBasket_Simscape_Optimizer/Subsystem1/Magnetic Torque//Force Generator3/Calculate Magnetic Force//Torque/Magnetic Torque ==
  r : Inport
  m1 : Inport  Port=2
  m2 : Inport  Port=3
  Add : Sum  Inputs=+-
  Constant : Constant  Value=-3
  Constant1 : Constant  Value=eye(3)
  Cross Product : matrix_library/Cross Product
  Display{,1..12} (13 alike) : Display
  Dot Product : DotProduct  OutDataTypeStr=Inherit: Inherit via internal rule
  Gain : Gain  Gain=Fixed.myu/(4*pi)
  Gain1 : Gain  Gain=3
  MatrixMultiply : Product  Multiplication=Matrix(*)
  MatrixMultiply1 : Product  Multiplication=Matrix(*)
  Normalize Vector : vrlib/Utilities/Normalize Vector  maxzero=0
  Normalize Vector1 : vrlib/Utilities/Normalize Vector  maxzero=0
  Power : Math  Operator=pow
  Product : Product
  Sqrt : Sqrt
  Transpose : Math  Operator=transpose
  Torque : Outport
  wires:
  Normalize Vector1/1 -> Display11/1
  Sqrt/1 -> Power/1  "|r|"
  Gain1/1 -> Display1/1, Add/1
  Product/1 -> Cross Product/2, Display/1
  MatrixMultiply1/1 -> Product/1, Display5/1
  Gain/1 -> Product/2, Display8/1
  m1/1 -> MatrixMultiply1/2, Display6/1
  Add/1 -> MatrixMultiply1/1, Display7/1
  Constant1/1 -> Add/2
  MatrixMultiply/1 -> Gain1/1, Display10/1
  Transpose/1 -> MatrixMultiply/2
  Normalize Vector/1 -> Display2/1, MatrixMultiply/1, Transpose/1, Display3/1  "r_hat"
  Power/1 -> Gain/1
  Constant/1 -> Power/2
  Dot Product/1 -> Sqrt/1
  r/1 -> Normalize Vector/1, Dot Product/1, Dot Product/2, Display9/1
  m2/1 -> Cross Product/1, Normalize Vector1/1, Display12/1
  Cross Product/1 -> Torque/1, Display4/1

== system MagneticBasket_Simscape_Optimizer/Subsystem1/Magnetic Torque//Force Generator4/Calculate Magnetic Force//Torque/Magnetic Force ==
  r : Inport
  m1 : Inport  Port=2
  m2 : Inport  Port=3
  Add : Sum  Inputs=+++
  Add2 : Sum  Inputs=+-
  Constant : Constant  Value=-4
  Display : Display
  Dot Product{1..5} (5 alike) : DotProduct  OutDataTypeStr=Inherit: Inherit via internal rule
  Gain : Gain  Gain=5
  Gain3 : Gain  Gain=3*Fixed.myu/(4*pi)
  Normalize Vector : vrlib/Utilities/Normalize Vector  maxzero=0
  Power : Math  Operator=pow
  Product{,1,4,6} (4 alike) : Product
  Sqrt : Sqrt
  Force : Outport
  wires:
  Dot Product1/1 -> Sqrt/1
  Constant/1 -> Power/2
  Power/1 -> Gain3/1
  Gain3/1 -> Product4/1  "3*myu_0/(4*pi*r^4)"
  Product4/1 -> Force/1
  r/1 -> Normalize Vector/1, Dot Product1/2, Dot Product1/1
  Normalize Vector/1 -> Product/1, Dot Product2/1, Dot Product4/1  "r_hat"
  m1/1 -> Dot Product3/1, Product1/2, Dot Product4/2  "m1"
  m2/1 -> Dot Product3/2, Dot Product2/2, Product6/2  "m2"
  Dot Product4/1 -> Product6/1, Dot Product5/1  "dot(m1,r_hat)"
  Dot Product2/1 -> Product1/1, Dot Product5/2  "dot(m2,r_hat)"
  Dot Product3/1 -> Add2/1  "dot(m1,m2)"
  Dot Product5/1 -> Gain/1
  Gain/1 -> Add2/2  "5 * dot(m1,r_hat) * dot(m2,r_hat)"
  Product1/1 -> Add/2
  Product6/1 -> Add/1
  Add/1 -> Product4/2
  Add2/1 -> Product/2
  Product/1 -> Add/3, Display/1
  Sqrt/1 -> Power/1

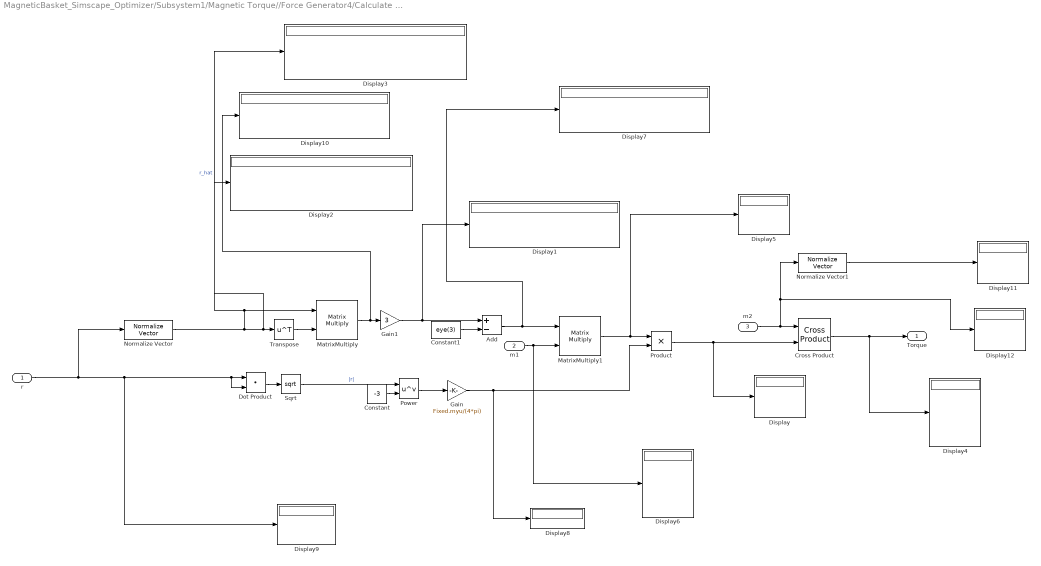
== system MagneticBasket_Simscape_Optimizer/Subsystem1/Magnetic Torque//Force Generator4/Calculate Magnetic Force//Torque/Magnetic Torque ==
  r : Inport
  m1 : Inport  Port=2
  m2 : Inport  Port=3
  Add : Sum  Inputs=+-
  Constant : Constant  Value=-3
  Constant1 : Constant  Value=eye(3)
  Cross Product : matrix_library/Cross Product
  Display{,1..12} (13 alike) : Display
  Dot Product : DotProduct  OutDataTypeStr=Inherit: Inherit via internal rule
  Gain : Gain  Gain=Fixed.myu/(4*pi)
  Gain1 : Gain  Gain=3
  MatrixMultiply : Product  Multiplication=Matrix(*)
  MatrixMultiply1 : Product  Multiplication=Matrix(*)
  Normalize Vector : vrlib/Utilities/Normalize Vector  maxzero=0
  Normalize Vector1 : vrlib/Utilities/Normalize Vector  maxzero=0
  Power : Math  Operator=pow
  Product : Product
  Sqrt : Sqrt
  Transpose : Math  Operator=transpose
  Torque : Outport
  wires:
  Cross Product/1 -> Display4/1, Torque/1
  m2/1 -> Display12/1, Normalize Vector1/1, Cross Product/1
  r/1 -> Display9/1, Dot Product/2, Dot Product/1, Normalize Vector/1
  Dot Product/1 -> Sqrt/1
  Constant/1 -> Power/2
  Power/1 -> Gain/1
  Normalize Vector/1 -> Display3/1, Transpose/1, MatrixMultiply/1, Display2/1  "r_hat"
  Transpose/1 -> MatrixMultiply/2
  MatrixMultiply/1 -> Display10/1, Gain1/1
  Constant1/1 -> Add/2
  Add/1 -> Display7/1, MatrixMultiply1/1
  m1/1 -> Display6/1, MatrixMultiply1/2
  Gain/1 -> Display8/1, Product/2
  MatrixMultiply1/1 -> Display5/1, Product/1
  Product/1 -> Display/1, Cross Product/2
  Gain1/1 -> Add/1, Display1/1
  Sqrt/1 -> Power/1  "|r|"
  Normalize Vector1/1 -> Display11/1

== system MagneticBasket_Simscape_Optimizer/Subsystem1/Magnetic Torque//Force Generator5/Calculate Magnetic Force//Torque/Magnetic Force ==
  r : Inport
  m1 : Inport  Port=2
  m2 : Inport  Port=3
  Add : Sum  Inputs=+++
  Add2 : Sum  Inputs=+-
  Constant : Constant  Value=-4
  Display : Display
  Dot Product{1..5} (5 alike) : DotProduct  OutDataTypeStr=Inherit: Inherit via internal rule
  Gain : Gain  Gain=5
  Gain3 : Gain  Gain=3*Fixed.myu/(4*pi)
  Normalize Vector : vrlib/Utilities/Normalize Vector  maxzero=0
  Power : Math  Operator=pow
  Product{,1,4,6} (4 alike) : Product
  Sqrt : Sqrt
  Force : Outport
  wires:
  Sqrt/1 -> Power/1
  Product/1 -> Display/1, Add/3
  Add2/1 -> Product/2
  Add/1 -> Product4/2
  Product6/1 -> Add/1
  Product1/1 -> Add/2
  Gain/1 -> Add2/2  "5 * dot(m1,r_hat) * dot(m2,r_hat)"
  Dot Product5/1 -> Gain/1
  Dot Product3/1 -> Add2/1  "dot(m1,m2)"
  Dot Product2/1 -> Dot Product5/2, Product1/1  "dot(m2,r_hat)"
  Dot Product4/1 -> Dot Product5/1, Product6/1  "dot(m1,r_hat)"
  m2/1 -> Product6/2, Dot Product2/2, Dot Product3/2  "m2"
  m1/1 -> Dot Product4/2, Product1/2, Dot Product3/1  "m1"
  Normalize Vector/1 -> Dot Product4/1, Dot Product2/1, Product/1  "r_hat"
  r/1 -> Dot Product1/1, Dot Product1/2, Normalize Vector/1
  Product4/1 -> Force/1
  Gain3/1 -> Product4/1  "3*myu_0/(4*pi*r^4)"
  Power/1 -> Gain3/1
  Constant/1 -> Power/2
  Dot Product1/1 -> Sqrt/1

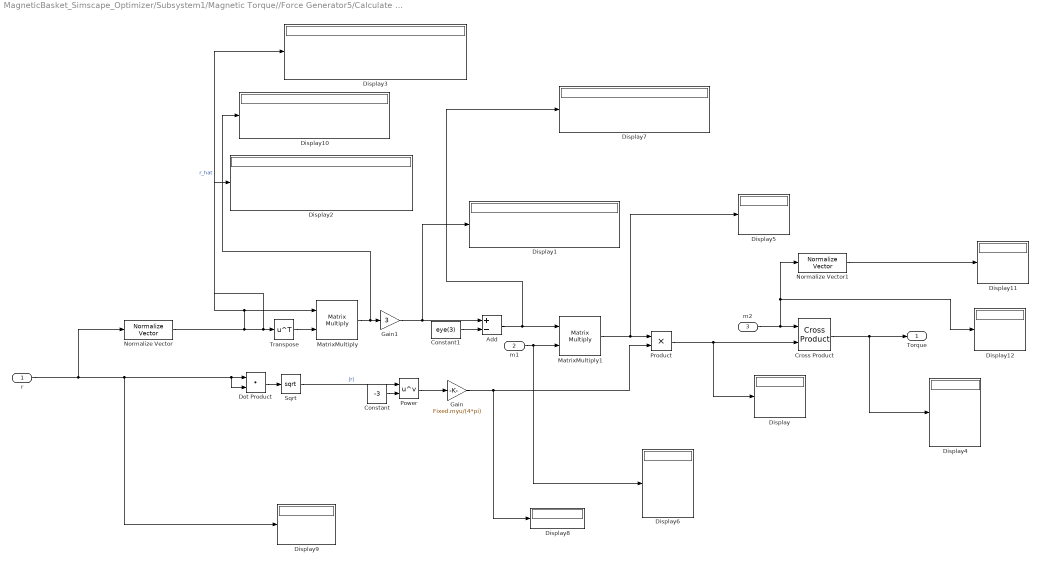
== system MagneticBasket_Simscape_Optimizer/Subsystem1/Magnetic Torque//Force Generator5/Calculate Magnetic Force//Torque/Magnetic Torque ==
  r : Inport
  m1 : Inport  Port=2
  m2 : Inport  Port=3
  Add : Sum  Inputs=+-
  Constant : Constant  Value=-3
  Constant1 : Constant  Value=eye(3)
  Cross Product : matrix_library/Cross Product
  Display{,1..12} (13 alike) : Display
  Dot Product : DotProduct  OutDataTypeStr=Inherit: Inherit via internal rule
  Gain : Gain  Gain=Fixed.myu/(4*pi)
  Gain1 : Gain  Gain=3
  MatrixMultiply : Product  Multiplication=Matrix(*)
  MatrixMultiply1 : Product  Multiplication=Matrix(*)
  Normalize Vector : vrlib/Utilities/Normalize Vector  maxzero=0
  Normalize Vector1 : vrlib/Utilities/Normalize Vector  maxzero=0
  Power : Math  Operator=pow
  Product : Product
  Sqrt : Sqrt
  Transpose : Math  Operator=transpose
  Torque : Outport
  wires:
  Normalize Vector1/1 -> Display11/1
  Sqrt/1 -> Power/1  "|r|"
  Gain1/1 -> Display1/1, Add/1
  Product/1 -> Cross Product/2, Display/1
  MatrixMultiply1/1 -> Product/1, Display5/1
  Gain/1 -> Product/2, Display8/1
  m1/1 -> MatrixMultiply1/2, Display6/1
  Add/1 -> MatrixMultiply1/1, Display7/1
  Constant1/1 -> Add/2
  MatrixMultiply/1 -> Gain1/1, Display10/1
  Transpose/1 -> MatrixMultiply/2
  Normalize Vector/1 -> Display2/1, MatrixMultiply/1, Transpose/1, Display3/1  "r_hat"
  Power/1 -> Gain/1
  Constant/1 -> Power/2
  Dot Product/1 -> Sqrt/1
  r/1 -> Normalize Vector/1, Dot Product/1, Dot Product/2, Display9/1
  m2/1 -> Cross Product/1, Normalize Vector1/1, Display12/1
  Cross Product/1 -> Torque/1, Display4/1

== system MagneticBasket_Simscape_Optimizer/Subsystem1/Magnetic Torque//Force Generator6/Calculate Magnetic Force//Torque/Magnetic Force ==
  r : Inport
  m1 : Inport  Port=2
  m2 : Inport  Port=3
  Add : Sum  Inputs=+++
  Add2 : Sum  Inputs=+-
  Constant : Constant  Value=-4
  Display : Display
  Dot Product{1..5} (5 alike) : DotProduct  OutDataTypeStr=Inherit: Inherit via internal rule
  Gain : Gain  Gain=5
  Gain3 : Gain  Gain=3*Fixed.myu/(4*pi)
  Normalize Vector : vrlib/Utilities/Normalize Vector  maxzero=0
  Power : Math  Operator=pow
  Product{,1,4,6} (4 alike) : Product
  Sqrt : Sqrt
  Force : Outport
  wires:
  Dot Product1/1 -> Sqrt/1
  Constant/1 -> Power/2
  Power/1 -> Gain3/1
  Gain3/1 -> Product4/1  "3*myu_0/(4*pi*r^4)"
  Product4/1 -> Force/1
  r/1 -> Normalize Vector/1, Dot Product1/2, Dot Product1/1
  Normalize Vector/1 -> Product/1, Dot Product2/1, Dot Product4/1  "r_hat"
  m1/1 -> Dot Product3/1, Product1/2, Dot Product4/2  "m1"
  m2/1 -> Dot Product3/2, Dot Product2/2, Product6/2  "m2"
  Dot Product4/1 -> Product6/1, Dot Product5/1  "dot(m1,r_hat)"
  Dot Product2/1 -> Product1/1, Dot Product5/2  "dot(m2,r_hat)"
  Dot Product3/1 -> Add2/1  "dot(m1,m2)"
  Dot Product5/1 -> Gain/1
  Gain/1 -> Add2/2  "5 * dot(m1,r_hat) * dot(m2,r_hat)"
  Product1/1 -> Add/2
  Product6/1 -> Add/1
  Add/1 -> Product4/2
  Add2/1 -> Product/2
  Product/1 -> Add/3, Display/1
  Sqrt/1 -> Power/1

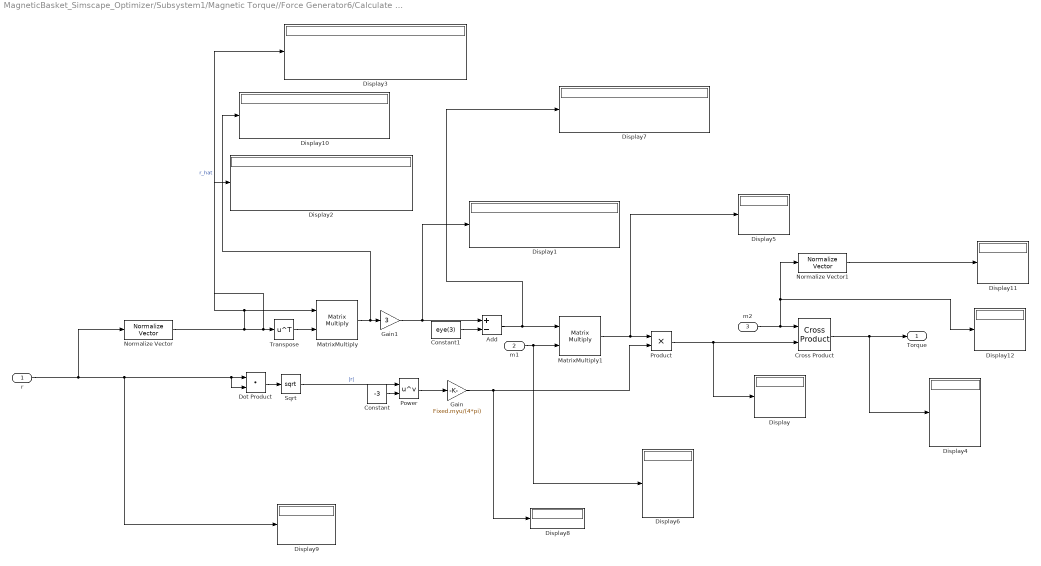
== system MagneticBasket_Simscape_Optimizer/Subsystem1/Magnetic Torque//Force Generator6/Calculate Magnetic Force//Torque/Magnetic Torque ==
  r : Inport
  m1 : Inport  Port=2
  m2 : Inport  Port=3
  Add : Sum  Inputs=+-
  Constant : Constant  Value=-3
  Constant1 : Constant  Value=eye(3)
  Cross Product : matrix_library/Cross Product
  Display{,1..12} (13 alike) : Display
  Dot Product : DotProduct  OutDataTypeStr=Inherit: Inherit via internal rule
  Gain : Gain  Gain=Fixed.myu/(4*pi)
  Gain1 : Gain  Gain=3
  MatrixMultiply : Product  Multiplication=Matrix(*)
  MatrixMultiply1 : Product  Multiplication=Matrix(*)
  Normalize Vector : vrlib/Utilities/Normalize Vector  maxzero=0
  Normalize Vector1 : vrlib/Utilities/Normalize Vector  maxzero=0
  Power : Math  Operator=pow
  Product : Product
  Sqrt : Sqrt
  Transpose : Math  Operator=transpose
  Torque : Outport
  wires:
  Cross Product/1 -> Display4/1, Torque/1
  m2/1 -> Display12/1, Normalize Vector1/1, Cross Product/1
  r/1 -> Display9/1, Dot Product/2, Dot Product/1, Normalize Vector/1
  Dot Product/1 -> Sqrt/1
  Constant/1 -> Power/2
  Power/1 -> Gain/1
  Normalize Vector/1 -> Display3/1, Transpose/1, MatrixMultiply/1, Display2/1  "r_hat"
  Transpose/1 -> MatrixMultiply/2
  MatrixMultiply/1 -> Display10/1, Gain1/1
  Constant1/1 -> Add/2
  Add/1 -> Display7/1, MatrixMultiply1/1
  m1/1 -> Display6/1, MatrixMultiply1/2
  Gain/1 -> Display8/1, Product/2
  MatrixMultiply1/1 -> Display5/1, Product/1
  Product/1 -> Display/1, Cross Product/2
  Gain1/1 -> Add/1, Display1/1
  Sqrt/1 -> Power/1  "|r|"
  Normalize Vector1/1 -> Display11/1

== system MagneticBasket_Simscape_Optimizer/Subsystem1/Magnetic Torque//Force Generator7/Calculate Magnetic Force//Torque/Magnetic Force ==
  r : Inport
  m1 : Inport  Port=2
  m2 : Inport  Port=3
  Add : Sum  Inputs=+++
  Add2 : Sum  Inputs=+-
  Constant : Constant  Value=-4
  Display : Display
  Dot Product{1..5} (5 alike) : DotProduct  OutDataTypeStr=Inherit: Inherit via internal rule
  Gain : Gain  Gain=5
  Gain3 : Gain  Gain=3*Fixed.myu/(4*pi)
  Normalize Vector : vrlib/Utilities/Normalize Vector  maxzero=0
  Power : Math  Operator=pow
  Product{,1,4,6} (4 alike) : Product
  Sqrt : Sqrt
  Force : Outport
  wires:
  Sqrt/1 -> Power/1
  Product/1 -> Display/1, Add/3
  Add2/1 -> Product/2
  Add/1 -> Product4/2
  Product6/1 -> Add/1
  Product1/1 -> Add/2
  Gain/1 -> Add2/2  "5 * dot(m1,r_hat) * dot(m2,r_hat)"
  Dot Product5/1 -> Gain/1
  Dot Product3/1 -> Add2/1  "dot(m1,m2)"
  Dot Product2/1 -> Dot Product5/2, Product1/1  "dot(m2,r_hat)"
  Dot Product4/1 -> Dot Product5/1, Product6/1  "dot(m1,r_hat)"
  m2/1 -> Product6/2, Dot Product2/2, Dot Product3/2  "m2"
  m1/1 -> Dot Product4/2, Product1/2, Dot Product3/1  "m1"
  Normalize Vector/1 -> Dot Product4/1, Dot Product2/1, Product/1  "r_hat"
  r/1 -> Dot Product1/1, Dot Product1/2, Normalize Vector/1
  Product4/1 -> Force/1
  Gain3/1 -> Product4/1  "3*myu_0/(4*pi*r^4)"
  Power/1 -> Gain3/1
  Constant/1 -> Power/2
  Dot Product1/1 -> Sqrt/1

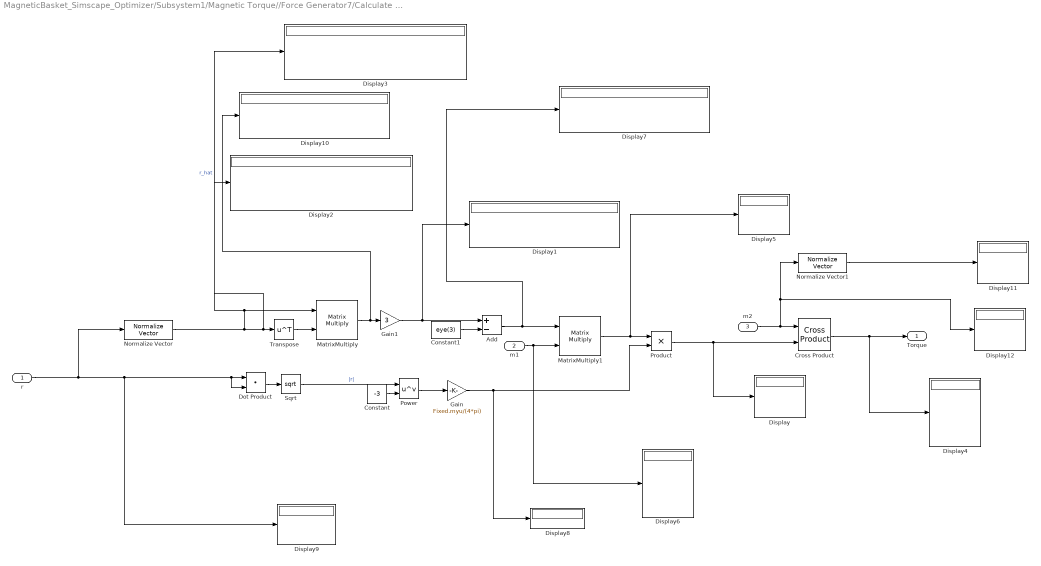
== system MagneticBasket_Simscape_Optimizer/Subsystem1/Magnetic Torque//Force Generator7/Calculate Magnetic Force//Torque/Magnetic Torque ==
  r : Inport
  m1 : Inport  Port=2
  m2 : Inport  Port=3
  Add : Sum  Inputs=+-
  Constant : Constant  Value=-3
  Constant1 : Constant  Value=eye(3)
  Cross Product : matrix_library/Cross Product
  Display{,1..12} (13 alike) : Display
  Dot Product : DotProduct  OutDataTypeStr=Inherit: Inherit via internal rule
  Gain : Gain  Gain=Fixed.myu/(4*pi)
  Gain1 : Gain  Gain=3
  MatrixMultiply : Product  Multiplication=Matrix(*)
  MatrixMultiply1 : Product  Multiplication=Matrix(*)
  Normalize Vector : vrlib/Utilities/Normalize Vector  maxzero=0
  Normalize Vector1 : vrlib/Utilities/Normalize Vector  maxzero=0
  Power : Math  Operator=pow
  Product : Product
  Sqrt : Sqrt
  Transpose : Math  Operator=transpose
  Torque : Outport
  wires:
  Normalize Vector1/1 -> Display11/1
  Sqrt/1 -> Power/1  "|r|"
  Gain1/1 -> Display1/1, Add/1
  Product/1 -> Cross Product/2, Display/1
  MatrixMultiply1/1 -> Product/1, Display5/1
  Gain/1 -> Product/2, Display8/1
  m1/1 -> MatrixMultiply1/2, Display6/1
  Add/1 -> MatrixMultiply1/1, Display7/1
  Constant1/1 -> Add/2
  MatrixMultiply/1 -> Gain1/1, Display10/1
  Transpose/1 -> MatrixMultiply/2
  Normalize Vector/1 -> Display2/1, MatrixMultiply/1, Transpose/1, Display3/1  "r_hat"
  Power/1 -> Gain/1
  Constant/1 -> Power/2
  Dot Product/1 -> Sqrt/1
  r/1 -> Normalize Vector/1, Dot Product/1, Dot Product/2, Display9/1
  m2/1 -> Cross Product/1, Normalize Vector1/1, Display12/1
  Cross Product/1 -> Torque/1, Display4/1
